simulink model "LookupTableND_5D_linear_clip"  (R2017b)
settings: Solver=FixedStepDiscrete  StartTime=0.0  StopTime=10.0  FixedStep=0.200000  RelTol=1e-3  EnableMultiTasking=on
settings Model: Creator=hbourbou  LastModifiedBy=hbourbou
settings DataIOCC: LimitDataPoints=on  SaveFormat=StructureWithTime
settings OptimizationCC: LifeSpan=inf
settings DebuggingCC: SFUnexpectedBacktrackingDiag=warning  SFNoUnconditionalDefaultTransitionDiag=warning  SFExecutionAtInitializationDiag=none
settings HardwareCC: ProdBitPerSizeT=32  ProdBitPerPtrDiffT=32  ProdWordSize=32  ProdHWDeviceType=Specified
settings ModelReferenceCC: PropagateSignalLabelsOutOfModel=off
settings CodeAppCC: StateflowObjectComments=on
settings GRTTargetCC: TargetLangStandard=C89/C90 (ANSI)
settings ConfigComp: CovMetricSettings=dw  CovHtmlReporting=on  CovSaveCumulativeToWorkspaceVar=on  CovSaveSingleToWorkspaceVar=on  CovExternalEMLEnable=off

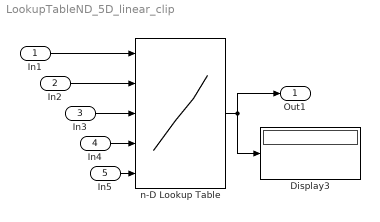
== system LookupTableND_5D_linear_clip ==
  In1 : Inport
  In2 : Inport  Port=2
  In3 : Inport  Port=3
  In4 : Inport  Port=4
  In5 : Inport  Port=5
  Display3 : Display
  n-D Lookup Table : Lookup_n-D  NumberOfTableDimensions=5  BreakpointsForDimension1=[1 7]  BreakpointsForDimension2="[2  5]"  BreakpointsForDimension3="[1  4]"  BreakpointsForDimension4=[1 2 5]  BreakpointsForDimension5=[1 3]  Table=cat(5,cat(4, cat(3, [9 2; 6 5], [7 1; 8 4]), cat(3, [3 5; 0 1], [5 6; 2 1]), cat(3, [1 2; 3 4], [4 3;2 1])),3*cat(4, cat(3, [9 2; 6 5], [7 1; 8 4]), cat(3, [3 5; 0 1], [5 6; 2 1]), cat(3, [1 2; 3 4], [4 3;2 1])))  ExtrapMethod=Clip  InternalRulePriority=Speed  RndMeth=Simplest  InputSameDT=on
  Out1 : Outport
  wires:
  n-D Lookup Table/1 -> Out1/1, Display3/1
  In1/1 -> n-D Lookup Table/1
  In4/1 -> n-D Lookup Table/4
  In3/1 -> n-D Lookup Table/3
  In2/1 -> n-D Lookup Table/2
  In5/1 -> n-D Lookup Table/5
